simulink model "CalculateFeedforwardVoltages"  (R2026a)
settings: Solver=FixedStepDiscrete
undefined symbols (not defined in the file): flux_d_FF, flux_q_FF, id_FF, iq_FF
settings Model: DataDictionary=TractionEmotorSoftwareArchInterfaceData.sldd  Creator=dakaihu  LastModifiedBy=dakaihu
settings OptimizationCC: GainParamInheritBuiltInType=on  UseFloatMulNetSlope=on  InlineInvariantSignals=on  NoFixptDivByZeroProtection=on  EfficientFloat2IntCast=on  LifeSpan=1
settings HardwareCC: ProdBitPerChar=16.0  ProdBitPerInt=16.0  ProdLargestAtomicInteger=Integer  ProdWordSize=16.0  ProdHWDeviceType=Texas Instruments->C2000
settings RTWCC: SystemTargetFile=ert.tlc  GenCodeOnly=on  Description=Embedded Coder
settings CodeAppCC: MaxIdLength=60.0  CustomSymbolStrGlobalVar=rt$N$M  CustomSymbolStrType=$N$M  CustomSymbolStrFcn=$N$M$F  CustomSymbolStrMacro=$N$M  ReqsInCode=on
settings ERTTargetCC: ERTFilePackagingFormat=CompactWithDataFile  GenerateSampleERTMain=on  IncludeMdlTerminateFcn=off  CombineSignalStateStructs=on  SuppressErrorStatus=on  SupportAbsoluteTime=off  SupportComplex=off

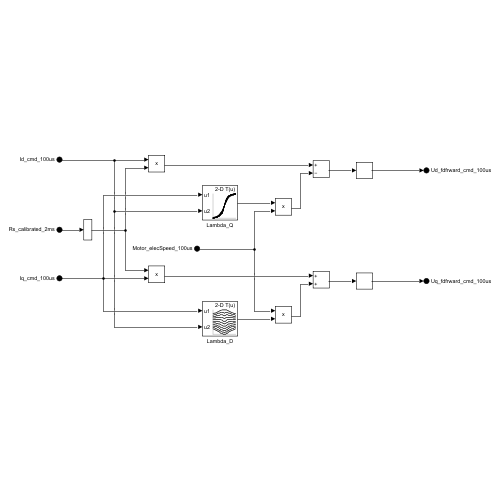
[thumbnail: Simulink's stored preview of the top-level diagram]
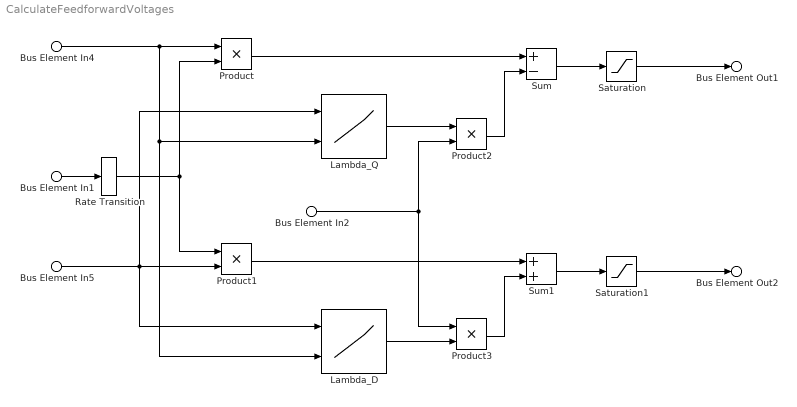
== system CalculateFeedforwardVoltages ==
  Bus Element In1 : Inport  PortName=Rs_calibrated_2ms
  Bus Element In5 : Inport  Port=2  PortName=Iq_cmd_100us
  Bus Element In2 : Inport  Port=3  PortName=Motor_elecSpeed_100us
  Bus Element In4 : Inport  Port=4  PortName=Id_cmd_100us
  Lambda_D : Lookup_n-D  BreakpointsForDimension1=iq_FF  BreakpointsForDimension2=id_FF  Table=flux_d_FF  InternalRulePriority=Speed  RndMeth=Simplest
      settings: InputPortMap=u0,u1
  Lambda_Q : Lookup_n-D  BreakpointsForDimension1=iq_FF  BreakpointsForDimension2=id_FF  Table=flux_q_FF  InternalRulePriority=Speed  RndMeth=Simplest
      settings: InputPortMap=u0,u1
  Product{,1..3} (4 alike) : Product
  Rate Transition : RateTransition  Deterministic=off  OutPortSampleTime=1e-4
  Saturation : Saturate  UpperLimit=250  LowerLimit=-250
  Saturation1 : Saturate  UpperLimit=250  LowerLimit=-250
  Sum : Sum  Inputs=+-
  Sum1 : Sum
  Bus Element Out1 : Outport  PortName=Ud_fdfrward_cmd_100us
  Bus Element Out2 : Outport  Port=2  PortName=Uq_fdfrward_cmd_100us
  wires:
  Bus Element In1/1 -> Rate Transition/1
  Bus Element In4/1 -> Lambda_D/2, Lambda_Q/2, Product/1
  Bus Element In5/1 -> Lambda_D/1, Product1/2, Lambda_Q/1
  Product/1 -> Sum/1
  Bus Element In2/1 -> Product3/1, Product2/2
  Lambda_Q/1 -> Product2/1
  Product2/1 -> Sum/2
  Sum/1 -> Saturation/1
  Lambda_D/1 -> Product3/2
  Saturation/1 -> Bus Element Out1/1
  Product1/1 -> Sum1/1
  Product3/1 -> Sum1/2
  Sum1/1 -> Saturation1/1
  Saturation1/1 -> Bus Element Out2/1
  Rate Transition/1 -> Product/2, Product1/1
